simulink model "hdlFrame_RGBFilter_3D_ForEach_SL"  (R2022b)
settings: Solver=FixedStepDiscrete  StartTime=0.0  StopTime=2  RelTol=1e-3
InitFcn:
  | R = 752;
  | C = 480;
  | redMax = 0;
  | greenMax = 255;
  | blueMax = 0;
undefined symbols (not defined in the file or in its folder): gray
libraries: visionsources x1
Description:
  | Sobel Edge Detection Using the MATLAB(R) Function Block
  | This example shows how to use HDL Coder(TM) to check,
  | generate, and verify HDL code for a Sobel Edge Detection
  | block built using the MATLAB Function block.
settings Model: FPTRunName=Active  Creator=The MathWorks, Inc.  LastModifiedBy=kkintali
settings SolverCC: AlgebraicLoopSolver=TrustRegion  MaxZcPerStep=1
settings DataIOCC: LimitDataPoints=on  SaveFormat=Array  SignalLogging=off  ReturnWorkspaceOutputs=off
settings OptimizationCC: BlockReduction=off  ConditionallyExecuteInputs=off  DefaultParameterBehavior=Inlined  ExpressionDepthLimit=2147483647  InitFltsAndDblsToZero=on  EfficientMapNaN2IntZero=off  LifeSpan=inf
settings DebuggingCC: AlgebraicLoopMsg=error  SaveWithParameterizedLinksMsg=none  UnderspecifiedInitializationDetection=Classic  MergeDetectMultiDrivingBlocksExec=none  SignalResolutionControl=TryResolveAllWithWarning  MultiTaskDSMMsg=warning  MultiTaskCondExecSysMsg=none  SingleTaskRateTransMsg=error  IntegerOverflowMsg=none  ParameterPrecisionLossMsg=none  FcnCallInpInsideContextMsg=warning  UnconnectedInputMsg=warning  UnconnectedOutputMsg=warning  UnconnectedLineMsg=warning  AllowSymbolicDim=off  StateNameClashWarn=warning  StrictBusMsg=ErrorOnBusTreatedAsVector  SFUnexpectedBacktrackingDiag=warning  SFNoUnconditionalDefaultTransitionDiag=warning  SFExecutionAtInitializationDiag=none  SFMachineParentedDataDiag=warning  IntegerSaturationMsg=none  ArithmeticOperatorsInVariantConditions=warning
settings HardwareCC: ProdBitPerPointer=32  ProdBitPerSizeT=32  ProdBitPerPtrDiffT=32  ProdLargestAtomicFloat=None  ProdIntDivRoundTo=Undefined  ProdEndianess=Unspecified  ProdWordSize=32  ProdHWDeviceType=ASIC/FPGA  TargetHWDeviceType=32-bit Generic  ProdEqTarget=off
settings ModelReferenceCC: EnableRefExpFcnMdlSchedulingChecks=on  PropagateSignalLabelsOutOfModel=off
settings SFSimCC: SimUseLocalCustomCode=off  CustomCodeUndefinedFunction=UseInterfaceOnly
settings RTWCC: PlatformDefinition=Embedded Code  RTWUseLocalCustomCode=off  DLArmComputeVersion=19.05
settings CodeAppCC: StateflowObjectComments=on
settings GRTTargetCC: TargetFcnLib=ansi_tfl_tmw.mat  TargetLangStandard=C89/C90 (ANSI)  CombineOutputUpdateFcns=off  GRTInterface=on
settings ConfigComp: CovMetricSettings=dw  CovSaveCumulativeToWorkspaceVar=on  CovSaveSingleToWorkspaceVar=on  CovExternalEMLEnable=off

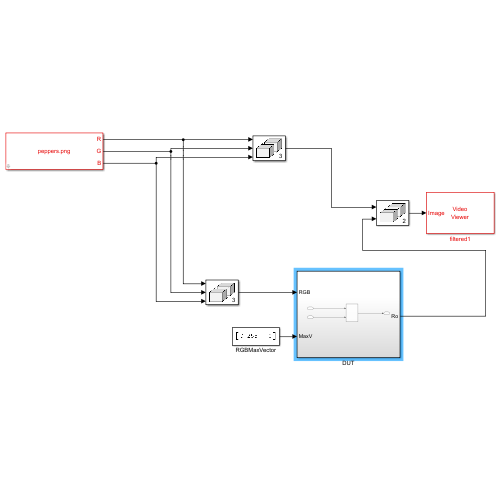
[thumbnail: Simulink's stored preview of the top-level diagram]
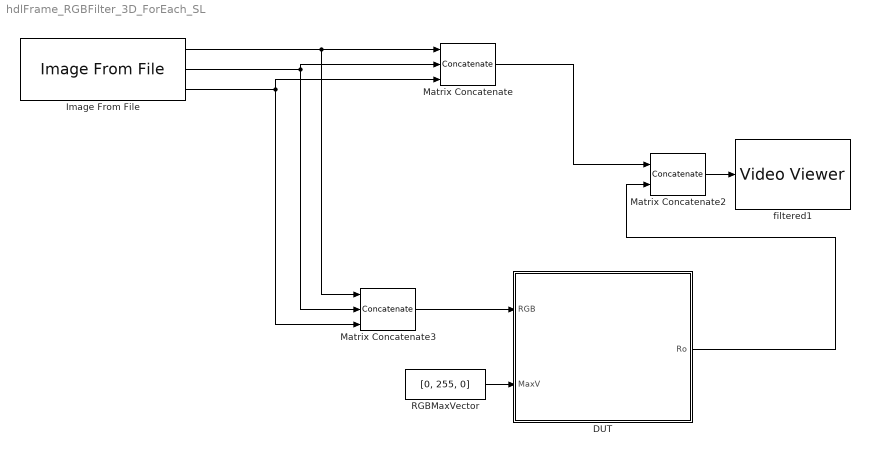
== system hdlFrame_RGBFilter_3D_ForEach_SL ==
  DUT : Subsystem
  Image From File : visionsources/Image From File  Tag=vipblks_nd  FileName=peppers.png  Ts=1  imagePorts=Separate color signals  OutPortLabels=R|G|B  ImageDataType=Inherit from input image  sdImageDataType=uint(8)  Signed=on  WordLength=16  FractionLengthMode=User-defined  FractionLength=15
  Matrix Concatenate : Concatenate  NumInputs=3  Mode=Multidimensional array  ConcatenateDimension=3
  Matrix Concatenate2 : Concatenate  Mode=Multidimensional array  ConcatenateDimension=2
  Matrix Concatenate3 : Concatenate  NumInputs=3  Mode=Multidimensional array  ConcatenateDimension=3
  RGBMaxVector : Constant  Value=[0, 255, 0]  OutDataTypeStr=uint8  SampleTime=-1
  filtered1 : VideoViewer  colormapValue=gray(256)  FigPos=[245 1292.66666666667 1280 622.666666666667]
  wires:
  RGBMaxVector/1 -> DUT/2(MaxV)
  Image From File/3 -> Matrix Concatenate3/3, Matrix Concatenate/3
  Image From File/2 -> Matrix Concatenate3/2, Matrix Concatenate/2
  Image From File/1 -> Matrix Concatenate3/1, Matrix Concatenate/1
  Matrix Concatenate/1 -> Matrix Concatenate2/1
  DUT/1(Ro) -> Matrix Concatenate2/2
  Matrix Concatenate2/1 -> filtered1/1
  Matrix Concatenate3/1 -> DUT/1(RGB)

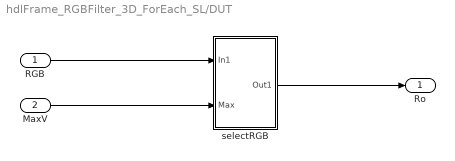
== system hdlFrame_RGBFilter_3D_ForEach_SL/DUT ==
  RGB : Inport
  MaxV : Inport  Port=2
  selectRGB : Subsystem
  Ro : Outport
  wires:
  MaxV/1 -> selectRGB/2(Max)
  RGB/1 -> selectRGB/1(In1)
  selectRGB/1(Out1) -> Ro/1

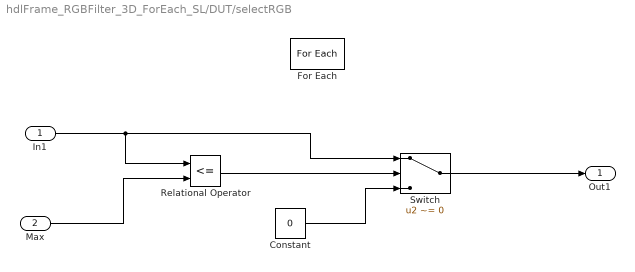
== system hdlFrame_RGBFilter_3D_ForEach_SL/DUT/selectRGB ==
  In1 : Inport  Partition=on  PartitionDimension=3  PartitionWidth=1  PartitionOffset=0
  Max : Inport  Port=2  Partition=on  PartitionDimension=1  PartitionWidth=1  PartitionOffset=0
  Constant : Constant  Value=0  OutDataTypeStr=uint8  SampleTime=-1
  For Each : ForEach  DisableCoverage=on
  Relational Operator : RelationalOperator  Operator=<=  OutDataTypeStr=boolean  RndMeth=Simplest  InputSameDT=off
  Switch : Switch  Criteria=u2 ~= 0  SaturateOnIntegerOverflow=off  InputSameDT=off
  Out1 : Outport  ConcatenationDimension=3
  wires:
  Constant/1 -> Switch/3
  In1/1 -> Switch/1, Relational Operator/1
  Relational Operator/1 -> Switch/2
  Max/1 -> Relational Operator/2
  Switch/1 -> Out1/1
